simulink model "InductionCookerStateFlow_HarnessInductionCookerS7"  (R2023a)
settings: Solver=FixedStepDiscrete  StartTime=0.0  StopTime=2000  FixedStep=0.1  RelTol=1e-3  EnableMultiTasking=on
settings Model: Creator=antonio  LastModifiedBy=anton
settings SolverCC: AlgebraicLoopSolver=TrustRegion  AutoInsertRateTranBlk=on
settings DataIOCC: LimitDataPoints=on
settings OptimizationCC: LifeSpan=inf
settings DebuggingCC: UnconnectedInputMsg=warning  UnconnectedOutputMsg=warning  UnconnectedLineMsg=warning  AllowSymbolicDim=off  SFUnexpectedBacktrackingDiag=warning  SFNoUnconditionalDefaultTransitionDiag=warning  SFExecutionAtInitializationDiag=none  ArithmeticOperatorsInVariantConditions=warning
settings ModelReferenceCC: EnableRefExpFcnMdlSchedulingChecks=on
settings SFSimCC: SimUseLocalCustomCode=off  CustomCodeUndefinedFunction=UseInterfaceOnly
settings RTWCC: RTWUseLocalCustomCode=off  DLArmComputeVersion=19.05
settings CodeAppCC: StateflowObjectComments=on
settings GRTTargetCC: TargetLangStandard=C89/C90 (ANSI)
settings ConfigComp: CovEnable=on  RecordCoverage=on  CovMetricSettings=dw  CovSaveCumulativeToWorkspaceVar=on  CovSaveSingleToWorkspaceVar=on  CovModelRefEnable=on

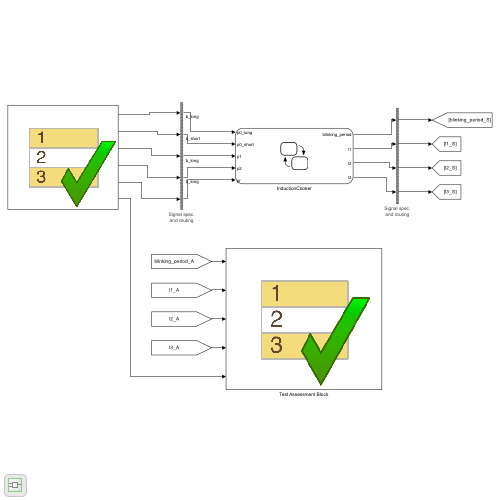
[thumbnail: Simulink's stored preview of the top-level diagram]
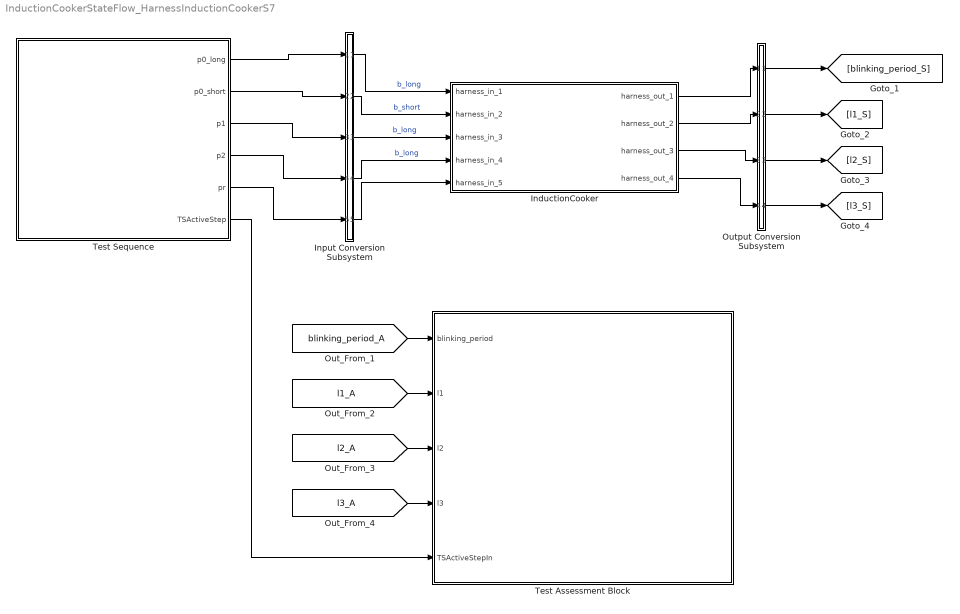
== system InductionCookerStateFlow_HarnessInductionCookerS7 ==
  InductionCooker : Subsystem  Tag=__SL_testing_harness_stub_
  Input Conversion Subsystem : Subsystem  Tag=__SLT_ICS__  Description=|
      | Signal spec.
      | and routing
      settings: AttributesFormatString=%<Description>
  Output Conversion Subsystem : Subsystem  Tag=__SLT_OCS__  Description=|
      | Signal spec.
      | and routing
      settings: AttributesFormatString=%<Description>
  Test Assessment Block : Test Sequence  Tag=__SLT_ASMT__  TreatAsAtomicUnit=on
  Test Sequence : Test Sequence  TreatAsAtomicUnit=on
  wires:
  [blinking_period_A] -> Test Assessment Block/1(blinking_period)
  [l1_A] -> Test Assessment Block/2(l1)
  [l2_A] -> Test Assessment Block/3(l2)
  [l3_A] -> Test Assessment Block/4(l3)
  Test Sequence/1(p0_long) -> Input Conversion Subsystem/1(Inport_1)
  Test Sequence/2(p0_short) -> Input Conversion Subsystem/2(Inport_2)
  Test Sequence/3(p1) -> Input Conversion Subsystem/3(Inport_3)
  Test Sequence/4(p2) -> Input Conversion Subsystem/4(Inport_4)
  Test Sequence/5(pr) -> Input Conversion Subsystem/5(Inport_5)
  Output Conversion Subsystem/1(Outport_1) -> [blinking_period_S]
  Output Conversion Subsystem/2(Outport_2) -> [l1_S]
  Output Conversion Subsystem/3(Outport_3) -> [l2_S]
  Output Conversion Subsystem/4(Outport_4) -> [l3_S]
  Test Sequence/6(TSActiveStep) -> Test Assessment Block/5(TSActiveStepIn)
  InductionCooker/1(harness_out_1) -> Output Conversion Subsystem/1(Inport_1)
  InductionCooker/2(harness_out_2) -> Output Conversion Subsystem/2(Inport_2)
  InductionCooker/3(harness_out_3) -> Output Conversion Subsystem/3(Inport_3)
  InductionCooker/4(harness_out_4) -> Output Conversion Subsystem/4(Inport_4)
  Input Conversion Subsystem/1(Outport_1) -> InductionCooker/1(harness_in_1)  "b_long"
  Input Conversion Subsystem/2(Outport_2) -> InductionCooker/2(harness_in_2)  "b_short"
  Input Conversion Subsystem/3(Outport_3) -> InductionCooker/3(harness_in_3)  "b_long"
  Input Conversion Subsystem/4(Outport_4) -> InductionCooker/4(harness_in_4)  "b_long"
  Input Conversion Subsystem/5(Outport_5) -> InductionCooker/5(harness_in_5)

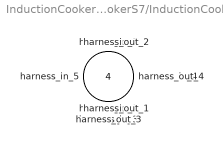
== system InductionCookerStateFlow_HarnessInductionCookerS7/InductionCooker ==
  harness_in_1 : Inport
  harness_in_2 : Inport  Port=2
  harness_in_3 : Inport  Port=3
  harness_in_4 : Inport  Port=4
  harness_in_5 : Inport  Port=5
  harness_out_1 : Outport
  harness_out_2 : Outport  Port=2
  harness_out_3 : Outport  Port=3
  harness_out_4 : Outport  Port=4

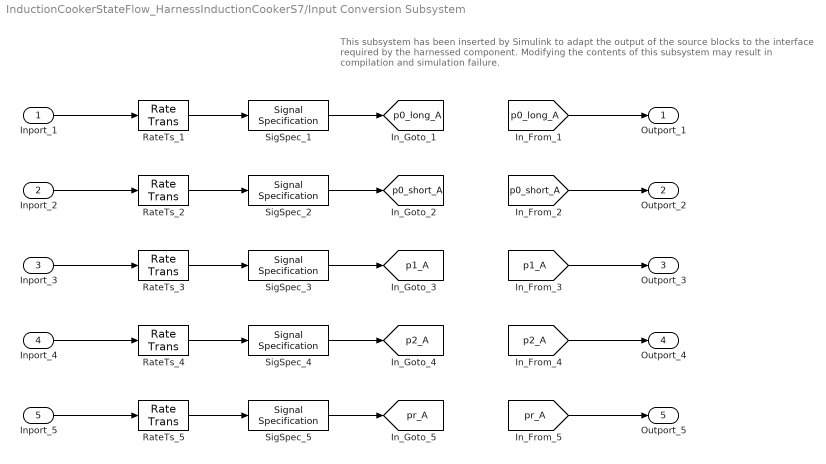
== system InductionCookerStateFlow_HarnessInductionCookerS7/Input Conversion Subsystem ==
  note: This subsystem has been inserted by Simulink to adapt the output of the source blocks to the interface required by the harnessed component.
      |  Modifying the contents of this subsystem may result in compilation and simulation failure.
  Inport_1 : Inport
  Inport_2 : Inport  Port=2
  Inport_3 : Inport  Port=3
  Inport_4 : Inport  Port=4
  Inport_5 : Inport  Port=5
  RateTs_{1..5} (5 alike) : RateTransition  OutPortSampleTime=0.1
  SigSpec_{1..5} (5 alike) : SignalSpecification  OutDataTypeStr=boolean  Dimensions=[1]  SampleTime=0.1
  Outport_1 : Outport
  Outport_2 : Outport  Port=2
  Outport_3 : Outport  Port=3
  Outport_4 : Outport  Port=4
  Outport_5 : Outport  Port=5
  tag scope: p0_long_A=global, p0_short_A=global, p1_A=global, p2_A=global, pr_A=global
  wires:
  [p0_long_A] -> Outport_1/1
  SigSpec_1/1 -> [p0_long_A]
  RateTs_1/1 -> SigSpec_1/1
  Inport_1/1 -> RateTs_1/1
  [p0_short_A] -> Outport_2/1
  SigSpec_2/1 -> [p0_short_A]
  RateTs_2/1 -> SigSpec_2/1
  Inport_2/1 -> RateTs_2/1
  [p1_A] -> Outport_3/1
  SigSpec_3/1 -> [p1_A]
  RateTs_3/1 -> SigSpec_3/1
  Inport_3/1 -> RateTs_3/1
  [p2_A] -> Outport_4/1
  SigSpec_4/1 -> [p2_A]
  RateTs_4/1 -> SigSpec_4/1
  Inport_4/1 -> RateTs_4/1
  [pr_A] -> Outport_5/1
  SigSpec_5/1 -> [pr_A]
  RateTs_5/1 -> SigSpec_5/1
  Inport_5/1 -> RateTs_5/1

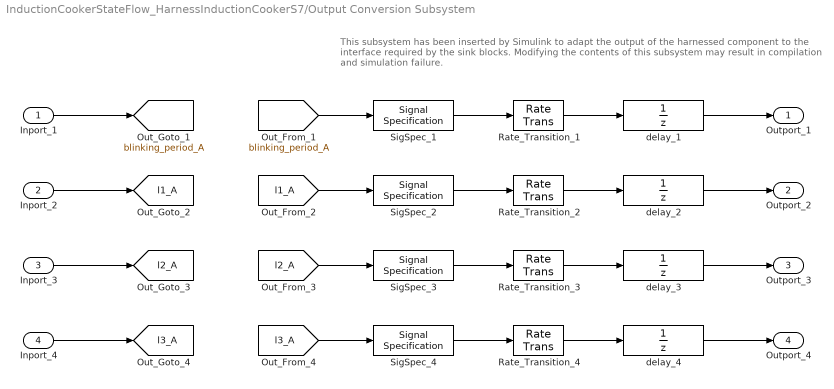
== system InductionCookerStateFlow_HarnessInductionCookerS7/Output Conversion Subsystem ==
  note: This subsystem has been inserted by Simulink to adapt the output of the harnessed component to the interface required by the sink blocks.
      |  Modifying the contents of this subsystem may result in compilation and simulation failure.
  Inport_1 : Inport
  Inport_2 : Inport  Port=2
  Inport_3 : Inport  Port=3
  Inport_4 : Inport  Port=4
  Rate_Transition_{1..4} (4 alike) : RateTransition  OutPortSampleTimeOpt=Inherit
  SigSpec_1 : SignalSpecification  OutDataTypeStr=uint32  Dimensions=[1]  SampleTime=0.1
  SigSpec_2 : SignalSpecification  OutDataTypeStr=boolean  Dimensions=[1]  SampleTime=0.1
  SigSpec_3 : SignalSpecification  OutDataTypeStr=boolean  Dimensions=[1]  SampleTime=0.1
  SigSpec_4 : SignalSpecification  OutDataTypeStr=boolean  Dimensions=[1]  SampleTime=0.1
  delay_{1..4} (4 alike) : UnitDelay  SampleTime=-1
  Outport_1 : Outport
  Outport_2 : Outport  Port=2
  Outport_3 : Outport  Port=3
  Outport_4 : Outport  Port=4
  tag scope: blinking_period_A=global, l1_A=global, l2_A=global, l3_A=global
  wires:
  Inport_1/1 -> [blinking_period_A]
  [blinking_period_A] -> SigSpec_1/1
  SigSpec_1/1 -> Rate_Transition_1/1
  Rate_Transition_1/1 -> delay_1/1
  delay_1/1 -> Outport_1/1
  Inport_2/1 -> [l1_A]
  [l1_A] -> SigSpec_2/1
  SigSpec_2/1 -> Rate_Transition_2/1
  Rate_Transition_2/1 -> delay_2/1
  delay_2/1 -> Outport_2/1
  Inport_3/1 -> [l2_A]
  [l2_A] -> SigSpec_3/1
  SigSpec_3/1 -> Rate_Transition_3/1
  Rate_Transition_3/1 -> delay_3/1
  delay_3/1 -> Outport_3/1
  Inport_4/1 -> [l3_A]
  [l3_A] -> SigSpec_4/1
  SigSpec_4/1 -> Rate_Transition_4/1
  Rate_Transition_4/1 -> delay_4/1
  delay_4/1 -> Outport_4/1

== stateflow chart InductionCookerStateFlow_HarnessInductionCookerS7/Test Assessment Block ==
  state Scenario_1
    state Run
      state VerifyInitS7
        verify(blinking_period == 0 & ~l1 & ~l2 & ~l3)
      state VerifyOnWithPotPresentS7
        verify(blinking_period == 0 & l1 & ~l2 & ~l3)
      state VerifyInactiveWithPotPresentS7
        verify(blinking_period == 0 & l1 & ~l2 & ~l3)
      state VerifyPowerIncreaseWithPotPresentS7
        verify(blinking_period == 0 & l1 & ~l2 & ~l3)
      state VerifyActive300WS7
        verify(blinking_period == 2000 & l1 & l2 & ~l3)
      state VerifyPowerIncreaseWithPotPresentAgainS7
        verify(blinking_period == 2000 & l1 & l2 & ~l3)
      state VerifyActive500WS7
        verify(blinking_period == 1000 & l1 & l2 & ~l3)
      state VerifyPowerIncreaseWithPotPresentAgain2S7
        verify(blinking_period == 1000 & l1 & l2 & ~l3)
      state VerifyActive1000WS7
        verify(blinking_period == 500 & l1 & l2 & ~l3)
      state VerifyPowerIncreaseWithPotPresentAgain3S7
        verify(blinking_period == 500 & l1 & l2 & ~l3)
      state VerifyActive1500WS7
        verify(blinking_period == 250 & l1 & l2 & ~l3)
      state VerifyPowerDecreaseWithPotPresentS7
        verify(blinking_period == 250 & l1 & l2 & ~l3)
      state VerifyActive1000WAgainS7
        verify(blinking_period == 500 & l1 & l2 & ~l3)
      state VerifyPowerDecreaseWithPotPresentAgainS7
        verify(blinking_period == 500 & l1 & l2 & ~l3)
      state VerifyActive500WAgainS7
        verify(blinking_period == 1000 & l1 & l2 & ~l3)
      state VerifyPowerDecreaseWithPotPresentAgain2S7
        verify(blinking_period == 1000 & l1 & l2 & ~l3)
      state VerifyActive300WAgainS7
        verify(blinking_period == 2000 & l1 & l2 & ~l3)
      state VerifyPowerDecreaseWithPotPresentAgain3S7
        verify(blinking_period == 2000 & l1 & l2 & ~l3)
      state VerifyPowerIncreaseWithPotPresentInactiveS7
        verify(blinking_period == 2000 & l1 & l2 & ~l3)
      state VerifyActive300WAgain2S7
        verify(blinking_period == 2000 & l1 & l2 & ~l3)
      state VerifyPowerDecreaseWithPotPresentAgain4S7
        verify(blinking_period == 2000 & l1 & l2 & ~l3)
      state VerifyInactiveWithPotPresentAgainS7
        verify(blinking_period == 0 & l1 & ~l2 & ~l3)
      state VerifyLongPressOffWithPotPresentS7
        verify(blinking_period == 0 & ~l1 & ~l2 & ~l3)
      state VerifyReleaseOffS7
        verify(blinking_period == 0 & ~l1 & ~l2 & ~l3)
      state step_1_2
      (default) -> (junction 897)
      Run -> (junction 897)
      (junction 897) -> (junction 898) [order 1] : [TSActiveStepIn == TSActiveStepEnumHInductionCooker.InitS7
          | ]
      (junction 898) -> VerifyInitS7 [order 1] : [~in(Scenario_1.Run.VerifyInitS7)]
      (junction 897) -> (junction 907) [order 2]
      (junction 898) -> (junction 901) [order 2]
      (junction 907) -> (junction 908) [order 1] : [TSActiveStepIn == TSActiveStepEnumHInductionCooker.OnWithPotPresentS7
          | ]
      (junction 908) -> VerifyOnWithPotPresentS7 [order 1] : [~in(Scenario_1.Run.VerifyOnWithPotPresentS7)]
      (junction 907) -> (junction 915) [order 2]
      (junction 908) -> (junction 911) [order 2]
      (junction 915) -> (junction 916) [order 1] : [TSActiveStepIn == TSActiveStepEnumHInductionCooker.InactiveWithPotPresentS7
          | ]
      (junction 916) -> VerifyInactiveWithPotPresentS7 [order 1] : [~in(Scenario_1.Run.VerifyInactiveWithPotPresentS7)]
      (junction 915) -> (junction 923) [order 2]
      (junction 916) -> (junction 919) [order 2]
      (junction 923) -> (junction 924) [order 1] : [TSActiveStepIn == TSActiveStepEnumHInductionCooker.PowerIncreaseWithPotPresentS7
          | ]
      (junction 924) -> VerifyPowerIncreaseWithPotPresentS7 [order 1] : [~in(Scenario_1.Run.VerifyPowerIncreaseWithPotPresentS7)]
      (junction 923) -> (junction 931) [order 2]
      (junction 924) -> (junction 927) [order 2]
      (junction 931) -> (junction 932) [order 1] : [TSActiveStepIn == TSActiveStepEnumHInductionCooker.Active300WS7
          | ]
      (junction 932) -> VerifyActive300WS7 [order 1] : [~in(Scenario_1.Run.VerifyActive300WS7)]
      (junction 931) -> (junction 939) [order 2]
      (junction 932) -> (junction 935) [order 2]
      (junction 939) -> (junction 940) [order 1] : [TSActiveStepIn == TSActiveStepEnumHInductionCooker.PowerIncreaseWithPotPresentAgainS7
          | ]
      (junction 940) -> VerifyPowerIncreaseWithPotPresentAgainS7 [order 1] : [~in(Scenario_1.Run.VerifyPowerIncreaseWithPotPresentAgainS7)]
      (junction 939) -> (junction 947) [order 2]
      (junction 940) -> (junction 943) [order 2]
      (junction 947) -> (junction 948) [order 1] : [TSActiveStepIn == TSActiveStepEnumHInductionCooker.Active500WS7
          | ]
      (junction 948) -> VerifyActive500WS7 [order 1] : [~in(Scenario_1.Run.VerifyActive500WS7)]
      (junction 947) -> (junction 982) [order 2]
      (junction 948) -> (junction 951) [order 2]
      (junction 982) -> (junction 983) [order 1] : [TSActiveStepIn == TSActiveStepEnumHInductionCooker.PowerIncreaseWithPotPresentAgain2S7
          | ]
      (junction 983) -> VerifyPowerIncreaseWithPotPresentAgain2S7 [order 1] : [~in(Scenario_1.Run.VerifyPowerIncreaseWithPotPresentAgain2S7)]
      (junction 982) -> (junction 991) [order 2]
      (junction 983) -> (junction 986) [order 2]
      (junction 991) -> (junction 992) [order 1] : [TSActiveStepIn == TSActiveStepEnumHInductionCooker.Active1000WS7
          | ]
      (junction 992) -> VerifyActive1000WS7 [order 1] : [~in(Scenario_1.Run.VerifyActive1000WS7)]
      (junction 991) -> (junction 1000) [order 2]
      (junction 992) -> (junction 995) [order 2]
      (junction 1000) -> (junction 1001) [order 1] : [TSActiveStepIn == TSActiveStepEnumHInductionCooker.PowerIncreaseWithPotPresentAgain3S7
          | ]
      (junction 1001) -> VerifyPowerIncreaseWithPotPresentAgain3S7 [order 1] : [~in(Scenario_1.Run.VerifyPowerIncreaseWithPotPresentAgain3S7)]
      (junction 1000) -> (junction 1009) [order 2]
      (junction 1001) -> (junction 1004) [order 2]
      (junction 1009) -> (junction 1010) [order 1] : [TSActiveStepIn == TSActiveStepEnumHInductionCooker.Active1500WS7
          | ]
      (junction 1010) -> VerifyActive1500WS7 [order 1] : [~in(Scenario_1.Run.VerifyActive1500WS7)]
      (junction 1009) -> (junction 1018) [order 2]
      (junction 1010) -> (junction 1013) [order 2]
      (junction 1018) -> (junction 1019) [order 1] : [TSActiveStepIn == TSActiveStepEnumHInductionCooker.PowerDecreaseWithPotPresentS7
          | ]
      (junction 1019) -> VerifyPowerDecreaseWithPotPresentS7 [order 1] : [~in(Scenario_1.Run.VerifyPowerDecreaseWithPotPresentS7)]
      (junction 1018) -> (junction 1027) [order 2]
      (junction 1019) -> (junction 1022) [order 2]
      (junction 1027) -> (junction 1028) [order 1] : [TSActiveStepIn == TSActiveStepEnumHInductionCooker.Active1000WAgainS7
          | ]
      (junction 1028) -> VerifyActive1000WAgainS7 [order 1] : [~in(Scenario_1.Run.VerifyActive1000WAgainS7)]
      (junction 1027) -> (junction 1036) [order 2]
      (junction 1028) -> (junction 1031) [order 2]
      (junction 1036) -> (junction 1037) [order 1] : [TSActiveStepIn == TSActiveStepEnumHInductionCooker.PowerDecreaseWithPotPresentAgainS7
          | ]
      (junction 1037) -> VerifyPowerDecreaseWithPotPresentAgainS7 [order 1] : [~in(Scenario_1.Run.VerifyPowerDecreaseWithPotPresentAgainS7)]
      (junction 1036) -> (junction 1045) [order 2]
      (junction 1037) -> (junction 1040) [order 2]
      (junction 1045) -> (junction 1046) [order 1] : [TSActiveStepIn == TSActiveStepEnumHInductionCooker.Active500WAgainS7
          | ]
      (junction 1046) -> VerifyActive500WAgainS7 [order 1] : [~in(Scenario_1.Run.VerifyActive500WAgainS7)]
      (junction 1045) -> (junction 1054) [order 2]
      (junction 1046) -> (junction 1049) [order 2]
      (junction 1054) -> (junction 1055) [order 1] : [TSActiveStepIn == TSActiveStepEnumHInductionCooker.PowerDecreaseWithPotPresentAgain2S7
          | ]
      (junction 1055) -> VerifyPowerDecreaseWithPotPresentAgain2S7 [order 1] : [~in(Scenario_1.Run.VerifyPowerDecreaseWithPotPresentAgain2S7)]
      (junction 1054) -> (junction 1063) [order 2]
      (junction 1055) -> (junction 1058) [order 2]
      (junction 1063) -> (junction 1064) [order 1] : [TSActiveStepIn == TSActiveStepEnumHInductionCooker.Active300WAgainS7
          | ]
      (junction 1064) -> VerifyActive300WAgainS7 [order 1] : [~in(Scenario_1.Run.VerifyActive300WAgainS7)]
      (junction 1063) -> (junction 1072) [order 2]
      (junction 1064) -> (junction 1067) [order 2]
      (junction 1072) -> (junction 1073) [order 1] : [TSActiveStepIn == TSActiveStepEnumHInductionCooker.PowerDecreaseWithPotPresentAgain3S7
          | ]
      (junction 1073) -> VerifyPowerDecreaseWithPotPresentAgain3S7 [order 1] : [~in(Scenario_1.Run.VerifyPowerDecreaseWithPotPresentAgain3S7)]
      (junction 1072) -> (junction 1081) [order 2]
      (junction 1073) -> (junction 1076) [order 2]
      (junction 1081) -> (junction 1082) [order 1] : [TSActiveStepIn == TSActiveStepEnumHInductionCooker.PowerIncreaseWithPotPresentInactiveS7
          | ]
      (junction 1082) -> VerifyPowerIncreaseWithPotPresentInactiveS7 [order 1] : [~in(Scenario_1.Run.VerifyPowerIncreaseWithPotPresentInactiveS7)]
      (junction 1081) -> (junction 1090) [order 2]
      (junction 1082) -> (junction 1085) [order 2]
      (junction 1090) -> (junction 1091) [order 1] : [TSActiveStepIn == TSActiveStepEnumHInductionCooker.Active300WAgain2S7
          | ]
      (junction 1091) -> VerifyActive300WAgain2S7 [order 1] : [~in(Scenario_1.Run.VerifyActive300WAgain2S7)]
      (junction 1090) -> (junction 1099) [order 2]
      (junction 1091) -> (junction 1094) [order 2]
      (junction 1099) -> (junction 1100) [order 1] : [TSActiveStepIn == TSActiveStepEnumHInductionCooker.PowerDecreaseWithPotPresentAgain4S7
          | ]
      (junction 1100) -> VerifyPowerDecreaseWithPotPresentAgain4S7 [order 1] : [~in(Scenario_1.Run.VerifyPowerDecreaseWithPotPresentAgain4S7)]
      (junction 1108) -> (junction 955) [order 2]
      (junction 1100) -> (junction 1103) [order 2]
      (junction 1108) -> (junction 1109) [order 1] : [TSActiveStepIn == TSActiveStepEnumHInductionCooker.InactiveWithPotPresentAgainS7
          | ]
      (junction 1109) -> VerifyInactiveWithPotPresentAgainS7 [order 1] : [~in(Scenario_1.Run.VerifyInactiveWithPotPresentAgainS7)]
      (junction 955) -> (junction 956) [order 1] : [TSActiveStepIn == TSActiveStepEnumHInductionCooker.LongPressOffWithPotPresentS7
          | ]
      (junction 956) -> VerifyLongPressOffWithPotPresentS7 [order 1] : [~in(Scenario_1.Run.VerifyLongPressOffWithPotPresentS7)]
      (junction 955) -> (junction 963) [order 2]
      (junction 956) -> (junction 959) [order 2]
      (junction 963) -> (junction 964) [order 1] : [TSActiveStepIn == TSActiveStepEnumHInductionCooker.ReleaseOffS7
          | ]
      (junction 964) -> VerifyReleaseOffS7 [order 1] : [~in(Scenario_1.Run.VerifyReleaseOffS7)]
      (junction 963) -> (junction 971) [order 2]
      (junction 964) -> (junction 967) [order 2]
      (junction 971) -> (junction 972)
      (junction 972) -> step_1_2 [order 1] : [~in(Scenario_1.Run.step_1_2)]
      (junction 972) -> (junction 975) [order 2]
      (junction 1109) -> (junction 1112) [order 2]
      (junction 1099) -> (junction 1108) [order 2]
    (default) -> Run
  (default) -> Scenario_1 : {assert(Active_Scenario_Index == 1,'The value of Scenario Parameter ''Active_Scenario_Index'' is not valid. Use the index of the scenario to specify it.')}
  data: blinking_period input uint32 size=[1]; l1 input boolean size=[1]; l2 input boolean size=[1]; l3 input boolean size=[1]; TSActiveStepIn input; Active_Scenario_Index parameter =1

== stateflow chart InductionCookerStateFlow_HarnessInductionCookerS7/Test Sequence ==
  settings: updateMethod=DISCRETE  sampleTime=0.1
  state Scenario_1
    state InitS7
      p0_long = true;
      p0_short = true;
      p1 = true;
      p2 = true;
      pr = false;
      settings: description=|
          | Condizione in cui tutti i pulsanti sono rilasciati e
          | la pentola è presente sul dispositivo.
    state OnWithPotPresentS7
      p0_long = true;
      p0_short = false;
      p1 = true;
      p2 = true;
      pr = false;
      settings: description=|
          | Condizione in cui il pulsante per l'accensione è
          | premuto, mentre tutti gli altri pulsanti sono
          | rilasciati e la pentola è presente sul dispositivo.
    state InactiveWithPotPresentS7
      p0_long = true;
      p0_short = true;
      p1 = true;
      p2 = true;
      pr = false;
      settings: description=|
          | Condizione in cui tutti i pulsanti sono rilasciati e la
          | pentola è presente sul dispositivo.
    state PowerIncreaseWithPotPresentS7
      p0_long = true;
      p0_short = true;
      p1 = false;
      p2 = true;
      pr =  false;
      settings: description=|
          | Condizione in cui il pulsante per l'aumento della
          | potenza è premuto per almeno 1 secondo, mentre
          | tutti gli altri pulsanti sono rilasciati e la pentola è
          | presente sul dispositivo.
    state Waiting300WS7
      p0_long = true;
      p0_short = true;
      p1 = true;
      p2 = true;
      pr =  false;
      settings: description=|
          | Condizione in cui tutti i pulsanti sono rilasciati
          | e la pentola è presente sul dispositivo.
          | Si attende che passino i 5 secondi per
          | l'effettivo cambio della potenza.
    state Active300WS7
      p0_long = true;
      p0_short = true;
      p1 = true;
      p2 = true;
      pr =  false;
      settings: description=|
          | Condizione in cui tutti i pulsanti sono rilasciati, la
          | pentola è presente sul dispositivo e quest'ultimo sta
          | erogando la potenza desiderata.
    state PowerIncreaseWithPotPresentAgainS7
      p0_long = true;
      p0_short = true;
      p1 = false;
      p2 = true;
      pr =  false;
      settings: description=|
          | Condizione in cui il pulsante per l'aumento della
          | potenza è premuto per almeno 1 secondo, mentre
          | tutti gli altri pulsanti sono rilasciati e la pentola è
          | presente sul dispositivo.
    state Waiting500WS7
      p0_long = true;
      p0_short = true;
      p1 = true;
      p2 = true;
      pr =  false;
      settings: description=|
          | Condizione in cui tutti i pulsanti sono rilasciati
          | e la pentola è presente sul dispositivo.
          | Si attende che passino i 5 secondi per
          | l'effettivo cambio della potenza.
    state Active500WS7
      p0_long = true;
      p0_short = true;
      p1 = true;
      p2 = true;
      pr =  false;
      settings: description=|
          | Condizione in cui si sta erogando la potenza
          | selezionata.
    state PowerIncreaseWithPotPresentAgain2S7
      p0_long = true;
      p0_short = true;
      p1 = false;
      p2 = true;
      pr =  false;
      settings: description=|
          | Condizione in cui il pulsante per l'aumento della
          | potenza è premuto per almeno 1 secondo, mentre
          | tutti gli altri pulsanti sono rilasciati e la pentola è
          | presente sul dispositivo.
    state Waiting1000WS7
      p0_long = true;
      p0_short = true;
      p1 = true;
      p2 = true;
      pr =  false;
      settings: description=|
          | Condizione in cui tutti i pulsanti sono rilasciati
          | e la pentola è presente sul dispositivo.
          | Si attende che passino i 5 secondi per
          | l'effettivo cambio della potenza.
    state Active1000WS7
      p0_long = true;
      p0_short = true;
      p1 = true;
      p2 = true;
      pr =  false;
      settings: description=|
          | Condizione in cui si sta erogando la potenza
          | selezionata.
    state PowerIncreaseWithPotPresentAgain3S7
      p0_long = true;
      p0_short = true;
      p1 = false;
      p2 = true;
      pr =  false;
      settings: description=|
          | Condizione in cui il pulsante per l'aumento della
          | potenza è premuto per almeno 1 secondo, mentre
          | tutti gli altri pulsanti sono rilasciati e la pentola è
          | presente sul dispositivo.
    state Waiting1500WS7
      p0_long = true;
      p0_short = true;
      p1 = true;
      p2 = true;
      pr =  false;
      settings: description=|
          | Condizione in cui tutti i pulsanti sono rilasciati
          | e la pentola è presente sul dispositivo.
          | Si attende che passino i 5 secondi per
          | l'effettivo cambio della potenza.
    state Active1500WS7
      p0_long = true;
      p0_short = true;
      p1 = true;
      p2 = true;
      pr =  false;
      settings: description=|
          | Condizione in cui si sta erogando la potenza
          | selezionata.
    state PowerDecreaseWithPotPresentS7
      p0_long = true;
      p0_short = true;
      p1 = true;
      p2 = false;
      pr =  false;
      settings: description=|
          | Condizione in cui il pulsante per la diminuzione della
          | potenza è premuto per almeno 1 secondo, mentre
          | tutti gli altri pulsanti sono rilasciati e la pentola è
          | presente sul dispositivo.
    state Waiting1000WAgainS7
      p0_long = true;
      p0_short = true;
      p1 = true;
      p2 = true;
      pr =  false;
      settings: description=|
          | Condizione in cui tutti i pulsanti sono rilasciati
          | e la pentola è presente sul dispositivo.
          | Si attende che passino i 5 secondi per
          | l'effettivo cambio della potenza.
    state Active1000WAgainS7
      p0_long = true;
      p0_short = true;
      p1 = true;
      p2 = true;
      pr =  false;
      settings: description=|
          | Condizione in cui si sta erogando la potenza
          | selezionata.
    state PowerDecreaseWithPotPresentAgainS7
      p0_long = true;
      p0_short = true;
      p1 = true;
      p2 = false;
      pr =  false;
      settings: description=|
          | Condizione in cui il pulsante per la diminuzione della
          | potenza è premuto per almeno 1 secondo, mentre
          | tutti gli altri pulsanti sono rilasciati e la pentola è
          | presente sul dispositivo.
    state Waiting500WAgainS7
      p0_long = true;
      p0_short = true;
      p1 = true;
      p2 = true;
      pr =  false;
      settings: description=|
          | Condizione in cui tutti i pulsanti sono rilasciati
          | e la pentola è presente sul dispositivo.
          | Si attende che passino i 5 secondi per
          | l'effettivo cambio della potenza.
    state Active500WAgainS7
      p0_long = true;
      p0_short = true;
      p1 = true;
      p2 = true;
      pr =  false;
      settings: description=|
          | Condizione in cui si sta erogando la potenza
          | selezionata.
    state PowerDecreaseWithPotPresentAgain2S7
      p0_long = true;
      p0_short = true;
      p1 = true;
      p2 = false;
      pr =  false;
      settings: description=|
          | Condizione in cui il pulsante per la diminuzione della
          | potenza è premuto per almeno 1 secondo, mentre
          | tutti gli altri pulsanti sono rilasciati e la pentola è
          | presente sul dispositivo.
    state Waiting300WAgainS7
      p0_long = true;
      p0_short = true;
      p1 = true;
      p2 = true;
      pr =  false;
      settings: description=|
          | Condizione in cui tutti i pulsanti sono rilasciati
          | e la pentola è presente sul dispositivo.
          | Si attende che passino i 5 secondi per
          | l'effettivo cambio della potenza.
    state Active300WAgainS7
      p0_long = true;
      p0_short = true;
      p1 = true;
      p2 = true;
      pr =  false;
      settings: description=|
          | Condizione in cui si sta erogando la potenza
          | selezionata.
    state PowerDecreaseWithPotPresentAgain3S7
      p0_long = true;
      p0_short = true;
      p1 = true;
      p2 = false;
      pr =  false;
      settings: description=|
          | Condizione in cui il pulsante per la diminuzione della
          | potenza è premuto per almeno 1 secondo, mentre
          | tutti gli altri pulsanti sono rilasciati e la pentola è
          | presente sul dispositivo.
    state WaitingInactiveS7
      p0_long = true;
      p0_short = true;
      p1 = true;
      p2 = true;
      pr =  false;
      settings: description=|
          | Condizione in cui tutti i pulsanti sono rilasciati
          | e la pentola è presente sul dispositivo.
          | Si attende che passino i 5 secondi per
          | l'effettivo cambio della potenza. Tuttavia,
          | se si preme il pulsante per la diminuzione della potenza
          | entro i 5 secondi previsti, il cambio effettivo avverà
          | rispetto all'ultima variazione richiesta.
    state PowerIncreaseWithPotPresentInactiveS7
      p0_long = true;
      p0_short = true;
      p1 = false;
      p2 = true;
      pr =  false;
      settings: description=|
          | Condizione in cui il pulsante per l'aumento della
          | potenza è premuto per almeno 1 secondo, mentre
          | tutti gli altri pulsanti sono rilasciati e la pentola è
          | presente sul dispositivo.
    state Waiting300WAgain2S7
      p0_long = true;
      p0_short = true;
      p1 = true;
      p2 = true;
      pr =  false;
      settings: description=|
          | Condizione in cui tutti i pulsanti sono rilasciati
          | e la pentola è presente sul dispositivo.
          | Si attende che passino i 5 secondi per
          | l'effettivo cambio della potenza.
    state Active300WAgain2S7
      p0_long = true;
      p0_short = true;
      p1 = true;
      p2 = true;
      pr =  false;
      settings: description=|
          | Condizione in cui si sta erogando la potenza
          | selezionata.
    state PowerDecreaseWithPotPresentAgain4S7
      p0_long = true;
      p0_short = true;
      p1 = true;
      p2 = false;
      pr =  false;
      settings: description=|
          | Condizione in cui il pulsante per la diminuzione della
          | potenza è premuto per almeno 1 secondo, mentre
          | tutti gli altri pulsanti sono rilasciati e la pentola è
          | presente sul dispositivo.
    state WaitingInactiveAgainS7
      p0_long = true;
      p0_short = true;
      p1 = true;
      p2 = true;
      pr =  false;
      settings: description=|
          | Condizione in cui tutti i pulsanti sono rilasciati
          | e la pentola è presente sul dispositivo.
          | Si attende che passino i 5 secondi per
          | l'effettiva disattivazione del fornello.
    state InactiveWithPotPresentAgainS7
      p0_long = true;
      p0_short = true;
      p1 = true;
      p2 = true;
      pr = false;
      settings: description=|
          | Condizione in cui il fornello è stato disattivato tramite
          | una variazione di potenza da 300W a 0W richiesta
          | tramite il pulsante di diminuzione.
    state LongPressOffWithPotPresentS7
      p0_long = false;
      p0_short = true;
      p1 = true;
      p2 = true;
      pr =  false;
      settings: description=|
          | Condizione in cui il pulsante per lo spegnimento
          | è premuto per almeno 1 secondo, mentre tutti gli
          | altri pulsanti sono rilasciati e la pentola è presente
          | sul dispositivo.
    state ReleaseOffS7
      p0_long = true;
      p0_short = true;
      p1 = true;
      p2 = true;
      pr =  false;
      settings: description=|
          | Ritorno alla condizione iniziale rilasciando il
          | pulsante di spegnimento.
    (default) -> InitS7
    InitS7 -> OnWithPotPresentS7 : [
        | true
        | ]
    OnWithPotPresentS7 -> InactiveWithPotPresentS7 : [
        | true
        | ]
    InactiveWithPotPresentS7 -> PowerIncreaseWithPotPresentS7 : [
        | true
        | ]
    PowerIncreaseWithPotPresentS7 -> Waiting300WS7 : [
        | true
        | ]
    Waiting300WS7 -> Active300WS7 : [
        | after(5, sec)
        | ]
    Active300WS7 -> PowerIncreaseWithPotPresentAgainS7 : [
        | true
        | ]
    PowerIncreaseWithPotPresentAgainS7 -> Waiting500WS7 : [
        | true
        | ]
    Waiting500WS7 -> Active500WS7 : [
        | after(5, sec)
        | ]
    Active500WS7 -> PowerIncreaseWithPotPresentAgain2S7 : [
        | after(8, sec)
        | ]
    PowerIncreaseWithPotPresentAgain2S7 -> Waiting1000WS7 : [
        | true
        | ]
    Waiting1000WS7 -> Active1000WS7 : [
        | after(5,sec)
        | ]
    Active1000WS7 -> PowerIncreaseWithPotPresentAgain3S7 : [
        | after(2,sec)
        | ]
    PowerIncreaseWithPotPresentAgain3S7 -> Waiting1500WS7 : [
        | true
        | ]
    Waiting1500WS7 -> Active1500WS7 : [
        | after(5,sec)
        | ]
    Active1500WS7 -> PowerDecreaseWithPotPresentS7 : [
        | after(2,sec)
        | ]
    PowerDecreaseWithPotPresentS7 -> Waiting1000WAgainS7 : [
        | true
        | ]
    Waiting1000WAgainS7 -> Active1000WAgainS7 : [
        | after(5,sec)
        | ]
    Active1000WAgainS7 -> PowerDecreaseWithPotPresentAgainS7 : [
        | after(2,sec)
        | ]
    PowerDecreaseWithPotPresentAgainS7 -> Waiting500WAgainS7 : [
        | true
        | ]
    Waiting500WAgainS7 -> Active500WAgainS7 : [
        | after(5,sec)
        | ]
    Active500WAgainS7 -> PowerDecreaseWithPotPresentAgain2S7 : [
        | after(2,sec)
        | ]
    PowerDecreaseWithPotPresentAgain2S7 -> Waiting300WAgainS7 : [
        | true
        | ]
    Waiting300WAgainS7 -> Active300WAgainS7 : [
        | after(5,sec)
        | ]
    Active300WAgainS7 -> PowerDecreaseWithPotPresentAgain3S7 : [
        | after(2,sec)
        | ]
    PowerDecreaseWithPotPresentAgain3S7 -> WaitingInactiveS7 : [
        | true
        | ]
    WaitingInactiveS7 -> PowerIncreaseWithPotPresentInactiveS7 : [
        | after(2,sec)
        | ]
    PowerIncreaseWithPotPresentInactiveS7 -> Waiting300WAgain2S7 : [
        | true
        | ]
    Waiting300WAgain2S7 -> Active300WAgain2S7 : [
        | after(5,sec)
        | ]
    Active300WAgain2S7 -> PowerDecreaseWithPotPresentAgain4S7 : [
        | after(2,sec)
        | ]
    PowerDecreaseWithPotPresentAgain4S7 -> WaitingInactiveAgainS7 : [
        | true
        | ]
    InactiveWithPotPresentAgainS7 -> LongPressOffWithPotPresentS7 : [
        | after(2,sec)
        | ]
    LongPressOffWithPotPresentS7 -> ReleaseOffS7 : [
        | true
        | ]
    WaitingInactiveAgainS7 -> InactiveWithPotPresentAgainS7 : [
        | after(5,sec)
        | ]
  (default) -> Scenario_1 : {assert(Active_Scenario_Index == 1,'The value of Scenario Parameter ''Active_Scenario_Index'' is not valid. Use the index of the scenario to specify it.')}
  data: p0_long output boolean size=[1]; p0_short output boolean size=[1]; p1 output boolean size=[1]; p2 output boolean size=[1]; pr output boolean size=[1]; TSActiveStep output Enum: TSActiveStepEnumHInductionCooker; Active_Scenario_Index parameter =1
